simulink model "Boat_model"  (Simulink 6.6)
settings: Solver=ode3  StartTime=0.0  StopTime=10.0  FixedStep=.1  RelTol=1e-3
libraries: simulink x7
settings Model: Creator=Administrator  LastModifiedBy=Administrator

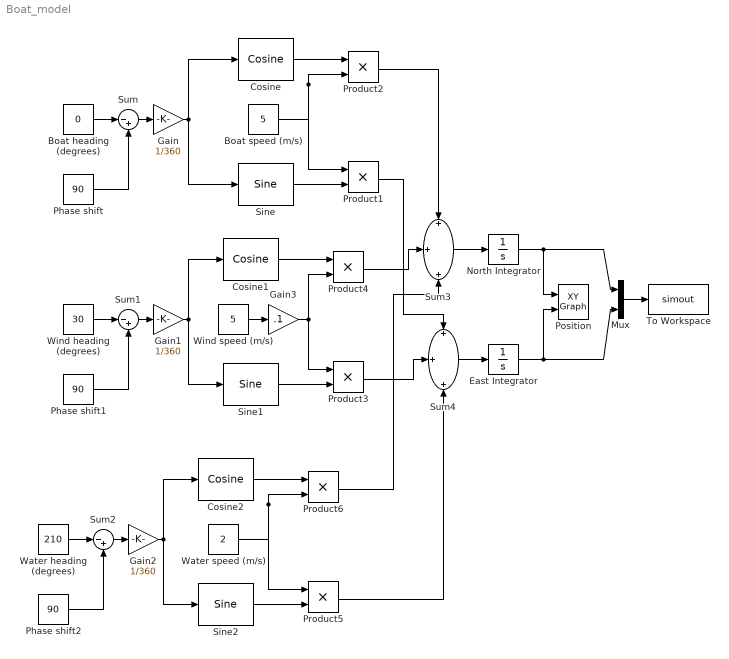
== system Boat_model ==
  Boat heading (degrees) : Constant  Value=0
  Boat speed (m/s) : Constant  Value=5
  Cosine : simulink/Lookup Tables/Cosine  SystemSampleTime=-1  Formula=cos(2*pi*u)  NumDataPoints=(2^5)+1  OutputWordLength=16
  Cosine1 : simulink/Lookup Tables/Cosine  SystemSampleTime=-1  Formula=cos(2*pi*u)  NumDataPoints=(2^5)+1  OutputWordLength=16
  Cosine2 : simulink/Lookup Tables/Cosine  SystemSampleTime=-1  Formula=cos(2*pi*u)  NumDataPoints=(2^5)+1  OutputWordLength=16
  East Integrator : Integrator
  Gain : Gain  Gain=1/360
  Gain1 : Gain  Gain=1/360
  Gain2 : Gain  Gain=1/360
  Gain3 : Gain  Gain=.1
  Mux : Mux  Inputs=2
  North Integrator : Integrator
  Phase shift : Constant  Value=90
  Phase shift1 : Constant  Value=90
  Phase shift2 : Constant  Value=90
  Position : simulink/Sinks/XY Graph  SystemSampleTime=-1  xmin=-100  xmax=100  ymin=-100  ymax=100  st=-1
  Product{1..6} (6 alike) : Product  RndMeth=Zero
  Sine : simulink/Lookup Tables/Sine  SystemSampleTime=-1  Formula=sin(2*pi*u)  NumDataPoints=(2^5)+1  OutputWordLength=16
  Sine1 : simulink/Lookup Tables/Sine  SystemSampleTime=-1  Formula=sin(2*pi*u)  NumDataPoints=(2^5)+1  OutputWordLength=16
  Sine2 : simulink/Lookup Tables/Sine  SystemSampleTime=-1  Formula=sin(2*pi*u)  NumDataPoints=(2^5)+1  OutputWordLength=16
  Sum : Sum  Inputs=|-+
  Sum1 : Sum  Inputs=|-+
  Sum2 : Sum  Inputs=|-+
  Sum3 : Sum  Inputs=+|+|+
  Sum4 : Sum  Inputs=+|+|+
  To Workspace : ToWorkspace  VariableName=simout  SampleTime=-1  SaveFormat=Structure
  Water heading (degrees) : Constant  Value=210
  Water speed (m/s) : Constant  Value=2
  Wind heading (degrees) : Constant  Value=30
  Wind speed (m/s) : Constant  Value=5
  wires:
  North Integrator/1 -> Position/1, Mux/1
  Boat speed (m/s)/1 -> Product1/1, Product2/2
  Cosine/1 -> Product2/1
  Gain/1 -> Cosine/1, Sine/1
  East Integrator/1 -> Position/2, Mux/2
  Sine/1 -> Product1/2
  Mux/1 -> To Workspace/1
  Sum/1 -> Gain/1
  Boat heading (degrees)/1 -> Sum/1
  Phase shift/1 -> Sum/2
  Cosine1/1 -> Product4/1
  Gain1/1 -> Cosine1/1, Sine1/1
  Product4/1 -> Sum3/2
  Sine1/1 -> Product3/2
  Product3/1 -> Sum4/2
  Sum1/1 -> Gain1/1
  Wind heading (degrees)/1 -> Sum1/1
  Phase shift1/1 -> Sum1/2
  Water speed (m/s)/1 -> Product5/1, Product6/2
  Cosine2/1 -> Product6/1
  Gain2/1 -> Cosine2/1, Sine2/1
  Product6/1 -> Sum3/3
  Sine2/1 -> Product5/2
  Product5/1 -> Sum4/3
  Sum2/1 -> Gain2/1
  Water heading (degrees)/1 -> Sum2/1
  Phase shift2/1 -> Sum2/2
  Sum3/1 -> North Integrator/1
  Sum4/1 -> East Integrator/1
  Product1/1 -> Sum4/1
  Product2/1 -> Sum3/1
  Wind speed (m/s)/1 -> Gain3/1
  Gain3/1 -> Product4/2, Product3/1
